simulink model "model_stationary"  (R2020a)
settings: Solver=ode23t  StartTime=0.0  StopTime=t_end  MaxStep=t_step_max  RelTol=solver_tol
values from neighbouring files (symbols this model uses):
  BACK_EMF_DECOUPLING_GAIN = 1    [load_params.m]
  c = 2/3    (= 0.666666666667)    [load_params.m]
  CROSS_COUPLING_DECOUPLING_GAIN = 1    [load_params.m]
  Ke = 0.1    [load_params.m]
  Ki_d = wb_i * R    (= 376.991118431)    [load_params.m]
  Ki_q = wb_i * R    (= 376.991118431)    [load_params.m]
  Kp_d = wb_i * Ld    (= 8.79645943005)    [load_params.m]
  Kp_q = wb_i * Lq    (= 6.28318530718)    [load_params.m]
  L0 = (Ld + Lq - (2*Llkg)) / 3    (= 0.00386666666667)    [load_params.m]
  lambda_pm = 0.1    [load_params.m]
  Ld = 7e-3    (= 0.007)    [load_params.m]
  Lg = (Ld - Lq) / 3    (= 0.000666666666667)    [load_params.m]
  Llkg = 0.2e-3    (= 0.0002)    [load_params.m]
  Lq = 5e-3    (= 0.005)    [load_params.m]
  OMEGA_E = 2*pi*60    (= 376.991118431)    [load_params.m]
  R = 0.3    [load_params.m]
settings Model: Creator=Nathan Petersen  LastModifiedBy=Nathan Petersen

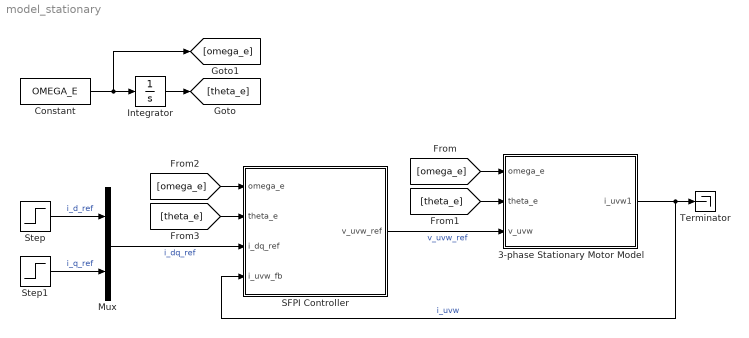
== system model_stationary ==
  3-phase Stationary Motor Model : Subsystem
  Constant : Constant  Value=OMEGA_E
  Integrator : Integrator
  Mux : Mux  Inputs=2
  SFPI Controller : Subsystem
  Step : Step  Time=0.1  SampleTime=0
  Step1 : Step  Time=0.2  SampleTime=0
  Terminator : Terminator
  wires:
  Step1/1 -> Mux/2  "i_q_ref"
  Step/1 -> Mux/1  "i_d_ref"
  Constant/1 -> [omega_e], Integrator/1
  Integrator/1 -> [theta_e]
  Mux/1 -> SFPI Controller/3(i_dq_ref)  "i_dq_ref"
  [omega_e] -> 3-phase Stationary Motor Model/1(omega_e)
  [theta_e] -> 3-phase Stationary Motor Model/2(theta_e)
  SFPI Controller/1(v_uvw_ref) -> 3-phase Stationary Motor Model/3(v_uvw)  "v_uvw_ref"
  3-phase Stationary Motor Model/1(i_uvw1) -> Terminator/1, SFPI Controller/4(i_uvw_fb)  "i_uvw"
  [omega_e] -> SFPI Controller/1(omega_e)
  [theta_e] -> SFPI Controller/2(theta_e)

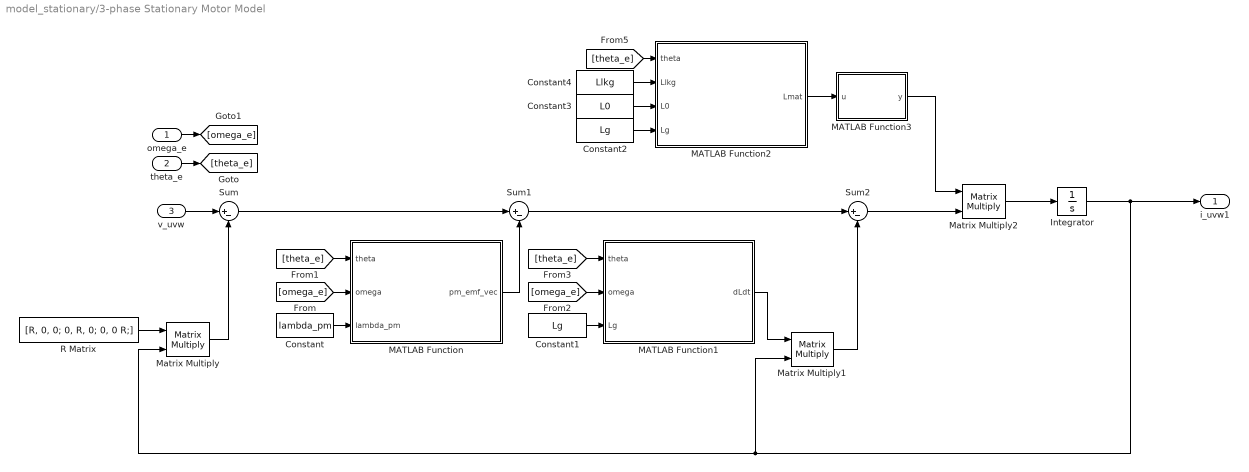
== system model_stationary/3-phase Stationary Motor Model ==
  omega_e : Inport
  theta_e : Inport  Port=2
  v_uvw : Inport  Port=3  PortDimensions=3
  Constant : Constant  Value=lambda_pm
  Constant1 : Constant  Value=Lg
  Constant2 : Constant  Value=Lg
  Constant3 : Constant  Value=L0
  Constant4 : Constant  Value=Llkg
  Integrator : Integrator
  MATLAB Function : MATLAB Function  TreatAsAtomicUnit=on
  MATLAB Function1 : MATLAB Function  TreatAsAtomicUnit=on
  MATLAB Function2 : MATLAB Function  TreatAsAtomicUnit=on
  MATLAB Function3 : MATLAB Function  TreatAsAtomicUnit=on
  Matrix Multiply : Product  Multiplication=Matrix(*)
  Matrix Multiply1 : Product  Multiplication=Matrix(*)
  Matrix Multiply2 : Product  Multiplication=Matrix(*)
  R Matrix : Constant  Value=[R, 0, 0; 0, R, 0; 0, 0 R;]
  Sum : Sum  Inputs=|+-
  Sum1 : Sum  Inputs=|+-
  Sum2 : Sum  Inputs=|+-
  i_uvw1 : Outport  PortDimensions=3
  wires:
  v_uvw/1 -> Sum/1
  R Matrix/1 -> Matrix Multiply/1
  Integrator/1 -> Matrix Multiply/2, Matrix Multiply1/2, i_uvw1/1
  Matrix Multiply/1 -> Sum/2
  Sum/1 -> Sum1/1
  MATLAB Function/1(pm_emf_vec) -> Sum1/2
  Sum1/1 -> Sum2/1
  MATLAB Function1/1(dLdt) -> Matrix Multiply1/1
  Matrix Multiply1/1 -> Sum2/2
  Matrix Multiply2/1 -> Integrator/1
  theta_e/1 -> [theta_e]
  omega_e/1 -> [omega_e]
  [theta_e] -> MATLAB Function/1(theta)
  [omega_e] -> MATLAB Function/2(omega)
  Constant/1 -> MATLAB Function/3(lambda_pm)
  [theta_e] -> MATLAB Function1/1(theta)
  [omega_e] -> MATLAB Function1/2(omega)
  Constant1/1 -> MATLAB Function1/3(Lg)
  [theta_e] -> MATLAB Function2/1(theta)
  Constant2/1 -> MATLAB Function2/4(Lg)
  Constant4/1 -> MATLAB Function2/2(Llkg)
  Constant3/1 -> MATLAB Function2/3(L0)
  Sum2/1 -> Matrix Multiply2/2
  MATLAB Function2/1(Lmat) -> MATLAB Function3/1(u)
  MATLAB Function3/1(y) -> Matrix Multiply2/1

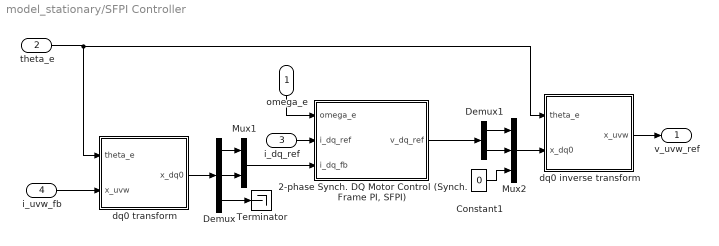
== system model_stationary/SFPI Controller ==
  omega_e : Inport
  theta_e : Inport  Port=2
  i_dq_ref : Inport  Port=3
  i_uvw_fb : Inport  Port=4
  "2-phase Synch. DQ Motor Control (Synch. Frame PI, SFPI)" : Subsystem
  Constant1 : Constant  Value=0
  Demux : Demux  Outputs=3
  Demux1 : Demux  Outputs=2
  Mux1 : Mux  Inputs=2
  Mux2 : Mux  Inputs=3
  Terminator : Terminator
  dq0 inverse transform : Subsystem
  dq0 transform : Subsystem
  v_uvw_ref : Outport
  wires:
  Demux/3 -> Terminator/1
  Demux/1 -> Mux1/1
  Demux/2 -> Mux1/2
  Demux1/1 -> Mux2/1
  Mux2/1 -> dq0 inverse transform/2(x_dq0)
  Demux1/2 -> Mux2/2
  Constant1/1 -> Mux2/3
  theta_e/1 -> dq0 transform/1(theta_e), dq0 inverse transform/1(theta_e)
  dq0 transform/1(x_dq0) -> Demux/1
  "2-phase Synch. DQ Motor Control (Synch. Frame PI, SFPI)"/1(v_dq_ref) -> Demux1/1
  Mux1/1 -> "2-phase Synch. DQ Motor Control (Synch. Frame PI, SFPI)"/3(i_dq_fb)
  omega_e/1 -> "2-phase Synch. DQ Motor Control (Synch. Frame PI, SFPI)"/1(omega_e)
  dq0 inverse transform/1(x_uvw) -> v_uvw_ref/1
  i_uvw_fb/1 -> dq0 transform/2(x_uvw)
  i_dq_ref/1 -> "2-phase Synch. DQ Motor Control (Synch. Frame PI, SFPI)"/2(i_dq_ref)

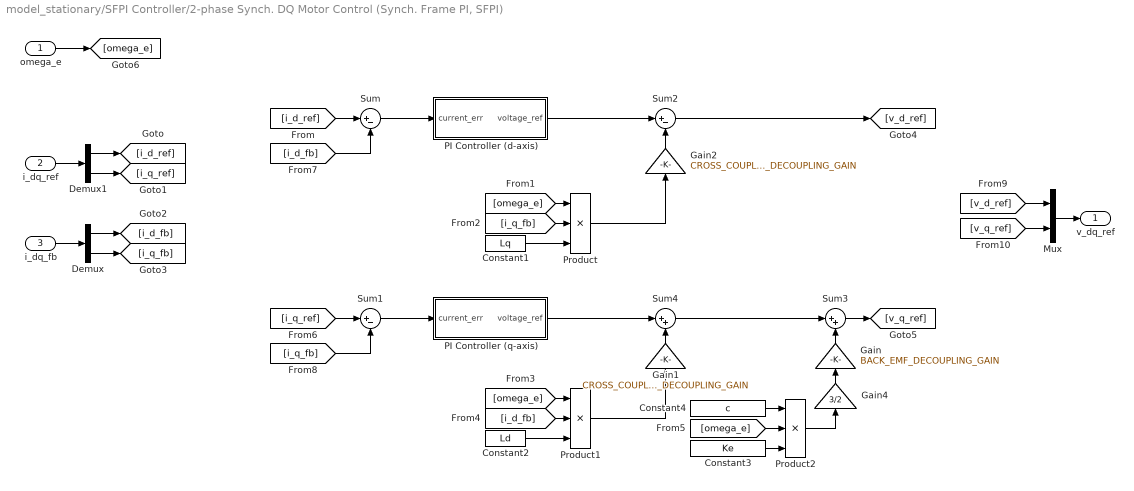
== system model_stationary/SFPI Controller/2-phase Synch. DQ Motor Control (Synch. Frame PI, SFPI) ==
  omega_e : Inport
  i_dq_ref : Inport  Port=2
  i_dq_fb : Inport  Port=3
  Constant1 : Constant  Value=Lq
  Constant2 : Constant  Value=Ld
  Constant3 : Constant  Value=Ke
  Constant4 : Constant  Value=c
  Demux : Demux  Outputs=2
  Demux1 : Demux  Outputs=2
  Gain : Gain  Gain=BACK_EMF_DECOUPLING_GAIN
  Gain1 : Gain  Gain=CROSS_COUPLING_DECOUPLING_GAIN
  Gain2 : Gain  Gain=CROSS_COUPLING_DECOUPLING_GAIN
  Gain4 : Gain  Gain=3/2
  Mux : Mux  Inputs=2
  PI Controller (d-axis) : Subsystem
  PI Controller (q-axis) : Subsystem
  Product : Product  Inputs=3
  Product1 : Product  Inputs=3
  Product2 : Product  Inputs=3
  Sum : Sum  Inputs=|+-
  Sum1 : Sum  Inputs=|+-
  Sum2 : Sum  Inputs=|+-
  Sum3 : Sum  Inputs=|++
  Sum4 : Sum  Inputs=|++
  v_dq_ref : Outport
  wires:
  Constant3/1 -> Product2/3
  Product/1 -> Gain2/1
  Sum/1 -> PI Controller (d-axis)/1(current_err)
  [omega_e] -> Product/1
  Sum2/1 -> [v_d_ref]
  PI Controller (d-axis)/1(voltage_ref) -> Sum2/1
  PI Controller (q-axis)/1(voltage_ref) -> Sum4/1
  [i_q_fb] -> Product/2
  Constant1/1 -> Product/3
  Constant4/1 -> Product2/1
  Product2/1 -> Gain4/1
  [i_d_fb] -> Product1/2
  Sum4/1 -> Sum3/1
  Constant2/1 -> Product1/3
  Product1/1 -> Gain1/1
  [omega_e] -> Product2/2
  Gain/1 -> Sum3/2
  Gain2/1 -> Sum2/2
  Gain1/1 -> Sum4/2
  Gain4/1 -> Gain/1
  Sum1/1 -> PI Controller (q-axis)/1(current_err)
  [omega_e] -> Product1/1
  Sum3/1 -> [v_q_ref]
  i_dq_fb/1 -> Demux/1
  i_dq_ref/1 -> Demux1/1
  Demux1/1 -> [i_d_ref]
  Demux1/2 -> [i_q_ref]
  Demux/2 -> [i_q_fb]
  Demux/1 -> [i_d_fb]
  [i_q_ref] -> Sum1/1
  [i_d_ref] -> Sum/1
  [i_d_fb] -> Sum/2
  [i_q_fb] -> Sum1/2
  [v_d_ref] -> Mux/1
  [v_q_ref] -> Mux/2
  Mux/1 -> v_dq_ref/1
  omega_e/1 -> [omega_e]

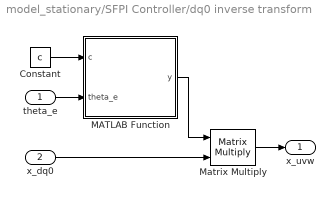
== system model_stationary/SFPI Controller/dq0 inverse transform ==
  theta_e : Inport
  x_dq0 : Inport  Port=2
  Constant : Constant  Value=c
  MATLAB Function : MATLAB Function  TreatAsAtomicUnit=on
  Matrix Multiply : Product  Multiplication=Matrix(*)
  x_uvw : Outport
  wires:
  Matrix Multiply/1 -> x_uvw/1
  MATLAB Function/1(y) -> Matrix Multiply/1
  x_dq0/1 -> Matrix Multiply/2
  theta_e/1 -> MATLAB Function/2(theta_e)
  Constant/1 -> MATLAB Function/1(c)

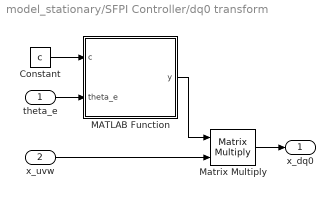
== system model_stationary/SFPI Controller/dq0 transform ==
  theta_e : Inport
  x_uvw : Inport  Port=2
  Constant : Constant  Value=c
  MATLAB Function : MATLAB Function  TreatAsAtomicUnit=on
  Matrix Multiply : Product  Multiplication=Matrix(*)
  x_dq0 : Outport
  wires:
  x_uvw/1 -> Matrix Multiply/2
  theta_e/1 -> MATLAB Function/2(theta_e)
  Constant/1 -> MATLAB Function/1(c)
  MATLAB Function/1(y) -> Matrix Multiply/1
  Matrix Multiply/1 -> x_dq0/1

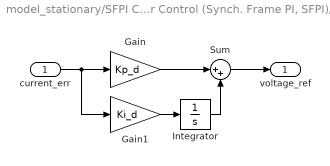
== system model_stationary/SFPI Controller/2-phase Synch. DQ Motor Control (Synch. Frame PI, SFPI)/PI Controller (d-axis) ==
  current_err : Inport
  Gain : Gain  Gain=Kp_d
  Gain1 : Gain  Gain=Ki_d
  Integrator : Integrator
  Sum : Sum  Inputs=|++
  voltage_ref : Outport
  wires:
  current_err/1 -> Gain1/1, Gain/1
  Gain/1 -> Sum/1
  Sum/1 -> voltage_ref/1
  Gain1/1 -> Integrator/1
  Integrator/1 -> Sum/2

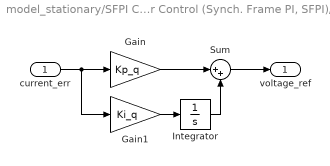
== system model_stationary/SFPI Controller/2-phase Synch. DQ Motor Control (Synch. Frame PI, SFPI)/PI Controller (q-axis) ==
  current_err : Inport
  Gain : Gain  Gain=Kp_q
  Gain1 : Gain  Gain=Ki_q
  Integrator : Integrator
  Sum : Sum  Inputs=|++
  voltage_ref : Outport
  wires:
  current_err/1 -> Gain1/1, Gain/1
  Gain/1 -> Sum/1
  Sum/1 -> voltage_ref/1
  Gain1/1 -> Integrator/1
  Integrator/1 -> Sum/2

== matlab function model_stationary/3-phase Stationary Motor Model/MATLAB Function3 ==
  data: u input; y output
function y = matinv(u)

y = inv(u);

== matlab function model_stationary/SFPI Controller/dq0 inverse transform/MATLAB Function ==
  data: c input; theta_e input; y output
function y = C_R_inv(c, theta_e)

y = (2/(3*c)) .* [
    cos(theta_e),             -sin(theta_e),           3*c/2;
    cos(theta_e + 4*pi/3),    -sin(theta_e + 4*pi/3),  3*c/2;
    cos(theta_e + 2*pi/3),    -sin(theta_e + 2*pi/3),  3*c/2;
];

end

== matlab function model_stationary/SFPI Controller/dq0 transform/MATLAB Function ==
  data: c input; theta_e input; y output
function y = C_R(c, theta_e)

y = c .* [
     cos(theta_e),  cos(theta_e - 2*pi/3),  cos(theta_e - 4*pi/3);
    -sin(theta_e), -sin(theta_e - 2*pi/3), -sin(theta_e - 4*pi/3);
          1/(3*c),                1/(3*c),                1/(3*c);
];

end

== matlab function model_stationary/3-phase Stationary Motor Model/MATLAB Function ==
  data: theta input; pm_emf_vec output; omega input; lambda_pm input
function pm_emf_vec = compute_pm_emf(theta, omega, lambda_pm)

pm_emf_vec = [
    (-lambda_pm * sin(theta) * omega);
    (lambda_pm * sin(theta + pi/3) * omega);
    (-lambda_pm * cos(theta + pi/6) * omega);
];

end

== matlab function model_stationary/3-phase Stationary Motor Model/MATLAB Function1 ==
  data: theta input; dLdt output; omega input; Lg input
function dLdt = compute_dL_dt(theta, omega, Lg)

dLdt = [
    -2*Lg*sin(2*theta)*omega,          2*Lg*sin(2*theta + 1/3*pi)*omega,  -2*Lg*cos(2*theta + 1/6*pi)*omega;
    2*Lg*sin(2*theta + 1/3*pi)*omega,  -2*Lg*cos(2*theta + 1/6*pi)*omega, -2*Lg*sin(2*theta)*omega;
    -2*Lg*cos(2*theta + 1/6*pi)*omega, -2*Lg*sin(2*theta)*omega,           2*Lg*sin(2*theta + 1/3*pi)*omega;
];

end

== matlab function model_stationary/3-phase Stationary Motor Model/MATLAB Function2 ==
  data: theta input; Lmat output; Llkg input; L0 input; Lg input
function Lmat = compute_Lmat(theta, Llkg, L0, Lg)

Lmat = [
    Llkg + L0 + Lg*cos(2*theta),       -1/2*L0 - Lg*cos(2*theta + 1/3*pi),       -1/2*L0 - Lg*sin(2*theta + 1/6*pi);
    -1/2*L0 - Lg*cos(2*theta + 1/3*pi),   Llkg + L0 - Lg*sin(2*theta + 1/6*pi),  -1/2*L0 + Lg*cos(2*theta);
    -1/2*L0 - Lg*sin(2*theta + 1/6*pi),  -1/2*L0 + Lg*cos(2*theta),                 Llkg + L0 - Lg*cos(2*theta + 1/3*pi);
];

end
